simulink model "UAV_Research_Environment"  (R2025a)
settings: Solver=ode23t  StartTime=0.0  StopTime=130  MaxStep=2e-3  RelTol=1e-4  AbsTol=1e-3  EnableMultiTasking=on
InitFcn:
  | skipInitialization = false;
  | 
  | if evalin('base', ...
  |         'exist(''CONTROLLER_TUNING_ACTIVE'',''var'')')
  | 
  |     skipInitialization = evalin('base', ...
  |         'logical(CONTROLLER_TUNING_ACTIVE)');
  | end
  | 
  | if ~skipInitialization
  | 
  |     icraControllerPrepared = false;
  | 
  |     hasICRAVariables = evalin('base', ...
  |         ['exist(''AUTOPILOT'',''var'') && ' ...
  |          'exist(''ICRA_ACTIVE_CONTROLLER'',''var'') && ' ...
  |          'exist(''ICRA_ACTIVE_RUN_ID'',''var'')']);
  | 
  |     if hasICRAVariables
  | 
  |         icraControllerPrepared = evalin('base', ...
  |             ['isstruct(AUTOPILOT) && ' ...
  |              'isfield(AUTOPILOT,''info'') && ' ...
  |              'isfield(AUTOPILOT.info,''ICRAControllerID'') && ' ...
  |              'strcmp(string(AUTOPILOT.info.ICRAControllerID), ' ...
  |                     'string(ICRA_ACTIVE_CONTROLLER))']);
  | 
  |     end
  | 
  |     if icraControllerPrepared
  |         skipInitialization = true;
  |     end
  | end
  | 
  | if ~skipInitialization
  | 
  |     mdl = bdroot;
  | 
  |     mdl_file = get_param(mdl, 'FileName');
  | 
  |     project_root = fileparts(mdl_file);
  | 
  |     init_file = fullfile(project_root, 'initialize_project.m');
  | 
  |     if exist(init_file, 'file')
  | 
  |         run(init_file);
  | 
  |     else
  | 
  |         error('initialize_project.m was not found in the model folder.');
  | 
  |     end
  | end
values from neighbouring files (symbols this model uses):
  A_UAV = struct()    [UAV_analytical.m]
  AUTOPILOT = struct()    [UAV_autopilot.m]
  B_UAV = struct()    [UAV_block.m]
  D = A_UAV.source.propeller_diameter_m    [UAV_analytical.m]    (also in plot_controller_results.m = permute(                  D,                  order); plot_estimator_results.m = permute(              D,              order); plot_mission_results.m = permute(                  D,                  order); plot_touchdown_diagnostics.m = permute(                  D,                  order))
  OPERATOR_MODE = OPERATOR_MODE_MANUAL    [initialize_project.m]    (also in uav_remote_gui.m = uint8(0))
  P_ENV = struct()    [Environment.m]
  P_UAV = struct()    [UAV_simscape.m]
  s = sin(angle)    [uav_remote_gui.m]
  SENSOR = struct()    [UAV_sensors.m]
  TRAJECTORY_CONFIG = struct()    [UAV_trajectories.m]
  TRAJECTORY_ID = uint8(          trajectoryIDNumeric)    [UAV_trajectories.m]
  X = reshape(                  D,                  nt,                  [])    [plot_controller_results.m]    (also in plot_estimator_results.m = reshape(              D,              nt,              []); plot_mission_results.m; plot_touchdown_diagnostics.m; plot_trajectory_3d.m)
  Y = absolutePlanNED(1,:)    [plot_trajectory_3d.m]    (also in uav_remote_gui.m = positionNED(:,1))
  Z = landedCGDown -          absolutePlanNED(3,:)    [plot_trajectory_3d.m]    (also in uav_remote_gui.m = landedCGDown-positionNED(:,3))
undefined symbols (not defined in the file or in its folder): Acceleration_ref, F, fractalcoef, Light, MIL, Position_ref, Velocity_ref, Yaw_ref, YawRate_ref
libraries: sm_lib x49, nesl_utility x29, fl_lib x17, slpidlib x16, simulink x14, ee_lib x5, sdl_lib x4, aerolibwind2 x3, aerolibatmos2 x2, sensorbarometerlib x1, sensorgpslib x1, mspsensorlib x1
(part 7 of 9)

== system UAV_Research_Environment/UAV Plant/UAV Physical [Simscape]/Motor ESC 3/Speed PI Control ==
  wCmd : Inport
  w : Inport  Port=2
  Gain : Gain  Gain=-1
  PI Controller : slpidlib/PID Controller  Controller=PI  Form=Parallel  TimeDomain=Continuous-time  UseExternalTs=off  SampleTime=-1  IntegratorMethod=Forward Euler  FilterMethod=Forward Euler  ControllerParametersSource=internal  P=P_UAV.drive.speed_pi.Kp  I=P_UAV.drive.speed_pi.Ki  UseKiTs=off  D=0.000001  UseExternalDerivativeSource=off  N=10000  UseFilter=on  TunerSelectOption=Transfer Function Based (PID Tuner App)  InitialConditionSource=internal  InitialConditionForIntegrator=0  InitialConditionForFilter=0  DifferentiatorICPrevScaledInput=0  ExternalReset=none  TrackingMode=off  Kt=1  LimitOutput=on  SatLimitsSource=internal  UpperSaturationLimit=P_UAV.drive.speed_pi.torque_limit_Nm  LowerSaturationLimit=-P_UAV.drive.speed_pi.torque_limit_Nm  LinearizeAsGain=on  AntiWindupMode=clamping  Kb=1  LimitIntegrator=off  UpperIntegratorSaturationLimit=inf  LowerIntegratorSaturationLimit=-inf  POutMin=[]  POutMax=[]  IOutMin=[]  IOutMax=[]  DOutMin=[]  DOutMax=[]  NOutMin=[]  NOutMax=[]  SumOutMin=[]  SumOutMax=[]  SaturationOutMin=[]  SaturationOutMax=[]  PParamMin=[]  PParamMax=[]  IParamMin=[]  IParamMax=[]  DParamMin=[]  DParamMax=[]  NParamMin=[]  NParamMax=[]  KbParamMin=[]  KbParamMax=[]  KtParamMin=[]  KtParamMax=[]  KbOutMin=[]  KbOutMax=[]  KtOutMin=[]  KtOutMax=[]  IntegratorOutMin=[]  IntegratorOutMax=[]  FilterOutMin=[]  FilterOutMax=[]  SumI1OutMin=[]  SumI1OutMax=[]  SumI2OutMin=[]  SumI2OutMax=[]  SumI3OutMin=[]  SumI3OutMax=[]  SumI4OutMin=[]  SumI4OutMax=[]  SumDOutMin=[]  SumDOutMax=[]  DifferentiatorOutMin=[]  DifferentiatorOutMax=[]  FilterDiffOutCoefMin=[]  FilterDiffOutCoefMax=[]  ReciprocalOutMin=[]  ReciprocalOutMax=[]  SumDenOutMin=[]  SumDenOutMax=[]  SumNumOutMin=[]  SumNumOutMax=[]  DivideOutMin=[]  DivideOutMax=[]  UdiffTsProdOutMin=[]  UdiffTsProdOutMax=[]  NTsProdOutMin=[]  NTsProdOutMax=[]  UintegralTsProdOutMin=[]  UintegralTsProdOutMax=[]  UngainTsProdOutMin=[]  UngainTsProdOutMax=[]  ClampingZeroOutDataTypeStr=Inherit: Inherit via back propagation  ClampingZeroOutMin=[]  ClampingZeroOutMax=[]  FilterDenConstantOutDataTypeStr=Inherit: Inherit via back propagation  FilterDenConstantOutMin=[]  FilterDenConstantOutMax=[]  PCopyOutDataTypeStr=Inherit: Inherit via back propagation  PCopyOutMin=[]  PCopyOutMax=[]  NCopyOutDataTypeStr=Inherit: Inherit via back propagation  NCopyOutMin=[]  NCopyOutMax=[]  IntegratorContinuousStateAttributes=''  IntegratorStateMustResolveToSignalObject=off  IntegratorRTWStateStorageClass=Auto  FilterContinuousStateAttributes=''  FilterStateMustResolveToSignalObject=off  FilterRTWStateStorageClass=Auto  ParallelPVariant=InternalParameters  IdealPVariant=Disabled  IVariant=InternalParameters  DVariant=Disabled  IntegratorVariant=Continuous  SatVariant=Enabled  AWVariant=ContClampingParallel  PCopyVariant=Disabled  TRVariant=Disabled  FdbkBlocksVariant=Forward  IdealPFdbkVariant=Disabled  SatFdbkVariant=Disabled  DerivativeFilterVariant=Disabled  NVariant=Disabled  NCopyVariant=Disabled_SignalSpec  FilterICVariant=Disabled  IntegratorICVariant=InternalICs  ExternalResetVariant=Disabled  TRSumVariant=Passthrough  SumFdbkVariant=Disabled  SumVariant=Sum_PI  TsampFilterVariant=InternalTs  TsampNgainVariant=Passthrough  TsampIntegralVariant=Disabled_SignalSpec  ExternalSaturationOutDataTypeStr=Inherit: Same as second input  DerivativeSourceVariant=Disabled  PreIntVariant=InternalPreInt
  Sum : Sum  Inputs=|+-
  TorqueCmd : Outport
  wires:
  wCmd/1 -> Gain/1
  Sum/1 -> PI Controller/1  "rad/s"
  w/1 -> Sum/2
  PI Controller/1 -> TorqueCmd/1  "N*m"
  Gain/1 -> Sum/1

== system UAV_Research_Environment/UAV Plant/UAV Physical [Simscape]/Motor ESC 4/Speed PI Control ==
  wCmd : Inport
  w : Inport  Port=2
  Gain : Gain  Gain=-1
  PI Controller : slpidlib/PID Controller  Controller=PI  Form=Parallel  TimeDomain=Continuous-time  UseExternalTs=off  SampleTime=-1  IntegratorMethod=Forward Euler  FilterMethod=Forward Euler  ControllerParametersSource=internal  P=P_UAV.drive.speed_pi.Kp  I=P_UAV.drive.speed_pi.Ki  UseKiTs=off  D=0.000001  UseExternalDerivativeSource=off  N=10000  UseFilter=on  TunerSelectOption=Transfer Function Based (PID Tuner App)  InitialConditionSource=internal  InitialConditionForIntegrator=0  InitialConditionForFilter=0  DifferentiatorICPrevScaledInput=0  ExternalReset=none  TrackingMode=off  Kt=1  LimitOutput=on  SatLimitsSource=internal  UpperSaturationLimit=P_UAV.drive.speed_pi.torque_limit_Nm  LowerSaturationLimit=-P_UAV.drive.speed_pi.torque_limit_Nm  LinearizeAsGain=on  AntiWindupMode=clamping  Kb=1  LimitIntegrator=off  UpperIntegratorSaturationLimit=inf  LowerIntegratorSaturationLimit=-inf  POutMin=[]  POutMax=[]  IOutMin=[]  IOutMax=[]  DOutMin=[]  DOutMax=[]  NOutMin=[]  NOutMax=[]  SumOutMin=[]  SumOutMax=[]  SaturationOutMin=[]  SaturationOutMax=[]  PParamMin=[]  PParamMax=[]  IParamMin=[]  IParamMax=[]  DParamMin=[]  DParamMax=[]  NParamMin=[]  NParamMax=[]  KbParamMin=[]  KbParamMax=[]  KtParamMin=[]  KtParamMax=[]  KbOutMin=[]  KbOutMax=[]  KtOutMin=[]  KtOutMax=[]  IntegratorOutMin=[]  IntegratorOutMax=[]  FilterOutMin=[]  FilterOutMax=[]  SumI1OutMin=[]  SumI1OutMax=[]  SumI2OutMin=[]  SumI2OutMax=[]  SumI3OutMin=[]  SumI3OutMax=[]  SumI4OutMin=[]  SumI4OutMax=[]  SumDOutMin=[]  SumDOutMax=[]  DifferentiatorOutMin=[]  DifferentiatorOutMax=[]  FilterDiffOutCoefMin=[]  FilterDiffOutCoefMax=[]  ReciprocalOutMin=[]  ReciprocalOutMax=[]  SumDenOutMin=[]  SumDenOutMax=[]  SumNumOutMin=[]  SumNumOutMax=[]  DivideOutMin=[]  DivideOutMax=[]  UdiffTsProdOutMin=[]  UdiffTsProdOutMax=[]  NTsProdOutMin=[]  NTsProdOutMax=[]  UintegralTsProdOutMin=[]  UintegralTsProdOutMax=[]  UngainTsProdOutMin=[]  UngainTsProdOutMax=[]  ClampingZeroOutDataTypeStr=Inherit: Inherit via back propagation  ClampingZeroOutMin=[]  ClampingZeroOutMax=[]  FilterDenConstantOutDataTypeStr=Inherit: Inherit via back propagation  FilterDenConstantOutMin=[]  FilterDenConstantOutMax=[]  PCopyOutDataTypeStr=Inherit: Inherit via back propagation  PCopyOutMin=[]  PCopyOutMax=[]  NCopyOutDataTypeStr=Inherit: Inherit via back propagation  NCopyOutMin=[]  NCopyOutMax=[]  IntegratorContinuousStateAttributes=''  IntegratorStateMustResolveToSignalObject=off  IntegratorRTWStateStorageClass=Auto  FilterContinuousStateAttributes=''  FilterStateMustResolveToSignalObject=off  FilterRTWStateStorageClass=Auto  ParallelPVariant=InternalParameters  IdealPVariant=Disabled  IVariant=InternalParameters  DVariant=Disabled  IntegratorVariant=Continuous  SatVariant=Enabled  AWVariant=ContClampingParallel  PCopyVariant=Disabled  TRVariant=Disabled  FdbkBlocksVariant=Forward  IdealPFdbkVariant=Disabled  SatFdbkVariant=Disabled  DerivativeFilterVariant=Disabled  NVariant=Disabled  NCopyVariant=Disabled_SignalSpec  FilterICVariant=Disabled  IntegratorICVariant=InternalICs  ExternalResetVariant=Disabled  TRSumVariant=Passthrough  SumFdbkVariant=Disabled  SumVariant=Sum_PI  TsampFilterVariant=InternalTs  TsampNgainVariant=Passthrough  TsampIntegralVariant=Disabled_SignalSpec  ExternalSaturationOutDataTypeStr=Inherit: Same as second input  DerivativeSourceVariant=Disabled  PreIntVariant=InternalPreInt
  Sum : Sum  Inputs=|+-
  TorqueCmd : Outport
  wires:
  Sum/1 -> PI Controller/1  "rad/s"
  w/1 -> Sum/2
  PI Controller/1 -> TorqueCmd/1  "N*m"
  Gain/1 -> Sum/1
  wCmd/1 -> Gain/1

== system UAV_Research_Environment/Autopilot/Flight Control/Main Controller/Horizontal Velocity Control/Subsystem ==
  CmdAcceleration_BodyXY : Inport
  Constant1 : Constant  Value=AUTOPILOT.horizontal.maxTilt_rad
  Constant2 : Constant  Value=-AUTOPILOT.horizontal.maxTilt_rad
  Gain : Gain  Gain=-1
  Gain1 : Gain  Gain=1 / AUTOPILOT.gravity.magnitude_m_s2
  Mux1 : Mux  Inputs=2
  Saturation Dynamic1 : simulink/Discontinuities/Saturation Dynamic  OutMin=[]  OutMax=[]  OutDataTypeStr=Inherit: Same as second input  OutDataType=fixdt(1, 16)  OutScaling=2^-10  DoSatur=off
  Selector2 : Selector  InputPortWidth=2  IndexOptions=Index vector (dialog)  Indices=1  OutputSizes=1
  Selector3 : Selector  InputPortWidth=2  IndexOptions=Index vector (dialog)  Indices=2  OutputSizes=1
  Trigonometric Function : Trigonometry  Operator=atan
  y : Outport
  wires:
  Trigonometric Function/1 -> Saturation Dynamic1/2  "CmdAttitude_raw"
  Mux1/1 -> Gain1/1
  Saturation Dynamic1/1 -> y/1
  Gain/1 -> Mux1/2  "MinusAx_cmd"
  CmdAcceleration_BodyXY/1 -> Selector3/1, Selector2/1
  Selector2/1 -> Gain/1  "Ax_cmd"
  Constant2/1 -> Saturation Dynamic1/3
  Gain1/1 -> Trigonometric Function/1
  Selector3/1 -> Mux1/1  "Ay_cmd"
  Constant1/1 -> Saturation Dynamic1/1

== matlab function UAV_Research_Environment/UAV Plant/UAV Analytical [ODEs]/Attitude Kinematics/Quaternion Kinematics ==
  data: Omega_body input; Q_dot output; Q input
function Q_dot = Quaternion_Kinematics(Omega_body,Q)

p = Omega_body(1);

q = Omega_body(2);

r = Omega_body(3);

Q_dot = 0.5 * [ ...
     0, -p, -q, -r; ...
     p,  0,  r, -q; ...
     q, -r,  0,  p; ...
     r,  q, -p,  0] * Q;

end

== matlab function UAV_Research_Environment/UAV Plant/UAV Analytical [ODEs]/Attitude Kinematics/Normalize Quaternion ==
  data: Q_raw input; Q output
function Q = Normalize_Quaternion(Q_raw)
%#codegen

n = sqrt(sum(Q_raw.^2));

if n > eps
    Q = Q_raw / n;
else
    Q = [1;0;0;0];
end

end

== matlab function UAV_Research_Environment/Live Telemetry/Telemetry_Pack ==
  data: t input; Telemetry output; Phase input; Active input; Complete input; Position_ref input; mode input; armed input; missionComplete input; Landed input; Position input; Euler input; MotorSpeeds input; MissionPlan input; TruePosition input; TrueEuler input; EstPosition input; NumWaypoints input
function Telemetry = Telemetry_Pack( ...
    t, ...
    Phase, ...
    Active, ...
    Complete, ...
    Position_ref, ...
    mode, ...
    armed, ...
    missionComplete, ...
    Landed, ...
    Position, ...
    Euler, ...
    MotorSpeeds, ...
    MissionPlan, ...
    TruePosition, ...
    TrueEuler, ...
    EstPosition, ...
    NumWaypoints)
maxWaypoints = ...
    size( ...
        MissionPlan, ...
        2);
genericTelemetryLength = ...
    59 + ...
    4*maxWaypoints;
Telemetry = ...
    zeros( ...
        genericTelemetryLength, ...
        1);
positionRefValid = ...
    numel(Position_ref) >= 3;
operationalPositionValid = ...
    numel(Position) >= 3;
operationalEulerValid = ...
    numel(Euler) >= 3;
motorSpeedsValid = ...
    numel(MotorSpeeds) >= 4;
truePositionValid = ...
    numel(TruePosition) >= 3;
trueEulerValid = ...
    numel(TrueEuler) >= 3;
estPositionValid = ...
    numel(EstPosition) >= 3;
missionPlanDimensionsValid = ...
    size(MissionPlan,1) == 4 && ...
    maxWaypoints >= 1;
numWaypointsRaw = ...
    double( ...
        NumWaypoints);
numWaypointsValid = ...
    isscalar(numWaypointsRaw) && ...
    isfinite(numWaypointsRaw) && ...
    numWaypointsRaw >= 1 && ...
    numWaypointsRaw <= maxWaypoints && ...
    abs( ...
        numWaypointsRaw - ...
        round(numWaypointsRaw)) < 1.0e-12;
if numWaypointsValid
    activeNumWaypoints = ...
        round( ...
            numWaypointsRaw);
else
    activeNumWaypoints = ...
        0.0;
end
Telemetry(1) = ...
    finiteScalarOrZero( ...
        t);
Telemetry(2) = ...
    finiteScalarOrZero( ...
        Phase);
Telemetry(3) = ...
    finiteScalarOrZero( ...
        Active);
Telemetry(4) = ...
    finiteScalarOrZero( ...
        Complete);
Telemetry(5) = ...
    finiteScalarOrZero( ...
        mode);
Telemetry(6) = ...
    finiteScalarOrZero( ...
        armed);
Telemetry(7) = ...
    finiteScalarOrZero( ...
        missionComplete);
Telemetry(8) = ...
    finiteScalarOrZero( ...
        Landed);
if positionRefValid
    Telemetry(9) = ...
        finiteScalarOrZero( ...
            Position_ref(1));
    Telemetry(10) = ...
        finiteScalarOrZero( ...
            Position_ref(2));
    Telemetry(11) = ...
        finiteScalarOrZero( ...
            Position_ref(3));
end
if operationalPositionValid
    Telemetry(12) = ...
        finiteScalarOrZero( ...
            Position(1));
    Telemetry(13) = ...
        finiteScalarOrZero( ...
            Position(2));
    Telemetry(14) = ...
        finiteScalarOrZero( ...
            Position(3));
end
legacyWaypointSlots = ...
    7;
if missionPlanDimensionsValid
    for k = 1:legacyWaypointSlots
        if k <= maxWaypoints
            Telemetry(14 + k) = ...
                finiteScalarOrZero( ...
                    MissionPlan(1,k));
            Telemetry(21 + k) = ...
                finiteScalarOrZero( ...
                    MissionPlan(2,k));
            Telemetry(28 + k) = ...
                finiteScalarOrZero( ...
                    MissionPlan(3,k));
            Telemetry(35 + k) = ...
                finiteScalarOrZero( ...
                    MissionPlan(4,k));
        end
    end
end
if operationalEulerValid
    Telemetry(43) = ...
        finiteScalarOrZero( ...
            Euler(1));
    Telemetry(44) = ...
        finiteScalarOrZero( ...
            Euler(2));
    Telemetry(45) = ...
        finiteScalarOrZero( ...
            Euler(3));
end
if motorSpeedsValid
    Telemetry(46) = ...
        finiteScalarOrZero( ...
            MotorSpeeds(1));
    Telemetry(47) = ...
        finiteScalarOrZero( ...
            MotorSpeeds(2));
    Telemetry(48) = ...
        finiteScalarOrZero( ...
            MotorSpeeds(3));
    Telemetry(49) = ...
        finiteScalarOrZero( ...
            MotorSpeeds(4));
end
if truePositionValid
    Telemetry(50) = ...
        finiteScalarOrZero( ...
            TruePosition(1));
    Telemetry(51) = ...
        finiteScalarOrZero( ...
            TruePosition(2));
    Telemetry(52) = ...
        finiteScalarOrZero( ...
            TruePosition(3));
end
if trueEulerValid
    Telemetry(53) = ...
        finiteScalarOrZero( ...
            TrueEuler(1));
    Telemetry(54) = ...
        finiteScalarOrZero( ...
            TrueEuler(2));
    Telemetry(55) = ...
        finiteScalarOrZero( ...
            TrueEuler(3));
end
if estPositionValid
    Telemetry(56) = ...
        finiteScalarOrZero( ...
            EstPosition(1));
    Telemetry(57) = ...
        finiteScalarOrZero( ...
            EstPosition(2));
    Telemetry(58) = ...
        finiteScalarOrZero( ...
            EstPosition(3));
end
Telemetry(59) = ...
    double( ...
        activeNumWaypoints);
northStartIndex = ...
    60;
eastStartIndex = ...
    60 + ...
    maxWaypoints;
downStartIndex = ...
    60 + ...
    2*maxWaypoints;
yawStartIndex = ...
    60 + ...
    3*maxWaypoints;
if missionPlanDimensionsValid && ...
        numWaypointsValid
    for k = 1:maxWaypoints
        if k <= activeNumWaypoints
            Telemetry( ...
                northStartIndex + k - 1) = ...
                finiteScalarOrZero( ...
                    MissionPlan(1,k));
            Telemetry( ...
                eastStartIndex + k - 1) = ...
                finiteScalarOrZero( ...
                    MissionPlan(2,k));
            Telemetry( ...
                downStartIndex + k - 1) = ...
                finiteScalarOrZero( ...
                    MissionPlan(3,k));
            Telemetry( ...
                yawStartIndex + k - 1) = ...
                finiteScalarOrZero( ...
                    MissionPlan(4,k));
        end
    end
end
end
function valueOut = finiteScalarOrZero(valueIn)
valueOut = ...
    double( ...
        valueIn);
if ~isfinite(valueOut)
    valueOut = ...
        0.0;
end
end

== stateflow chart UAV_Research_Environment/Autopilot/Flight Management/Mode Logic ==
  state Disarmed
    entry:
    mode = 1;
    armed = false;
    reset = true;
    missionComplete = false;
  state ArmedIdle
    entry:
    mode = 2;
    armed = true;
    reset = false;
    missionComplete = false;
  state TrajectoryMode
    entry:
    mode = 6;
    armed = true;
    reset = false;
    missionComplete = false;
  state LandingHold
    entry:
    mode = 6;
    armed = true;
    reset = false;
    missionComplete = true;
  state NavFailsafe
    entry:
    mode = 7;
    armed = true;
    reset = false;
    missionComplete = false;
  state FailsafeLanded
    entry:
    mode = 2;
    armed = true;
    reset = false;
    missionComplete = false;
  state TouchdownSettle
    entry:
    mode = 2;
    armed = true;
    reset = false;
    missionComplete = true;
  state LandedArmed
    entry:
    mode = 2;
    armed = true;
    reset = false;
    missionComplete = true;
  (default) -> Disarmed : {lastRunRequestID = uint32(0);}
  ArmedIdle -> TrajectoryMode [order 2] : [NavValid && RunTrajectoryRequestID ~= lastRunRequestID]
      | {lastRunRequestID = RunTrajectoryRequestID;}
  Disarmed -> ArmedIdle : [ArmCommand && NavValid]
  ArmedIdle -> Disarmed [order 1] : [~ArmCommand]
  TrajectoryMode -> Disarmed [order 1] : [~ArmCommand]
  LandedArmed -> TrajectoryMode [order 2] : [NavValid && RunTrajectoryRequestID ~= lastRunRequestID]
      | {lastRunRequestID = RunTrajectoryRequestID;}
  TrajectoryMode -> NavFailsafe [order 2] : [~NavValid]
  TrajectoryMode -> LandingHold [order 3] : [Complete]
  LandedArmed -> Disarmed [order 1] : [~ArmCommand]
  TouchdownSettle -> Disarmed [order 2] : [~ArmCommand]
  FailsafeLanded -> Disarmed : [~ArmCommand]
  NavFailsafe -> Disarmed [order 2] : [~ArmCommand]
  LandingHold -> Disarmed [order 1] : [~ArmCommand]
  LandingHold -> NavFailsafe [order 2] : [~NavValid]
  LandingHold -> TouchdownSettle [order 3] : [TouchdownCandidate]
  NavFailsafe -> FailsafeLanded [order 1] : [Landed]
  TouchdownSettle -> LandedArmed [order 1] : [Landed]
  data: mode output double size=1; armed output boolean size=1; reset output boolean size=1; missionComplete output boolean size=1; Complete input boolean; ArmCommand input boolean; RunTrajectoryRequestID input uint32; lastRunRequestID local uint32; Landed input boolean; TouchdownCandidate input boolean size=1; NavValid input boolean size=1

== matlab function UAV_Research_Environment/Autopilot/Flight Control/Error Computation/Wrap Yaw Error ==
  data: YawErrorRaw input; YawError output
function YawError = Wrap_Yaw_Error(YawErrorRaw)
%#codegen

YawError = atan2( ...
    sin(YawErrorRaw), ...
    cos(YawErrorRaw));

end

== matlab function UAV_Research_Environment/UAV Plant/UAV Analytical [ODEs]/Ground Contact/Ground_Contact_Model ==
  data: p_ned input; F_ground_body output; v_ned input; R_BN input; Omega_body input; Tau_ground_body output; UAV_CONTACT parameter
function [F_ground_body, Tau_ground_body] = ...
    Ground_Contact_Model( ...
        p_ned, ...
        v_ned, ...
        R_BN, ...
        Omega_body, ...
        UAV_CONTACT)
F_ground_body = ...
    zeros(3,1);
Tau_ground_body = ...
    zeros(3,1);
kGround = ...
    UAV_CONTACT.stiffness_N_m;
cGround = ...
    UAV_CONTACT.damping_N_s_m;
muStatic = ...
    UAV_CONTACT.static_friction;
muDynamic = ...
    UAV_CONTACT.dynamic_friction;
vCritical = ...
    UAV_CONTACT.critical_velocity_m_s;
if vCritical < 1e-6
    vCritical = ...
        1e-6;
end
groundDown = ...
    UAV_CONTACT.ground_down_m;
for i = 1:4
    r_body = [ ...
        UAV_CONTACT.arm_body_m(i,1);
        UAV_CONTACT.arm_body_m(i,2);
        UAV_CONTACT.arm_body_m(i,3)];
    r_ned = ...
        R_BN * r_body;
    p_contact_ned = ...
        p_ned + r_ned;
    v_rot_body = ...
        cross( ...
            Omega_body, ...
            r_body);
    v_rot_ned = ...
        R_BN * v_rot_body;
    v_contact_ned = ...
        v_ned + ...
        v_rot_ned;
    penetration = ...
        p_contact_ned(3) - ...
        groundDown;
    if penetration > 0.0
        penetrationRate = ...
            v_contact_ned(3);
        normalForce = ...
            kGround * penetration + ...
            cGround * penetrationRate;
        if normalForce < 0.0
            normalForce = ...
                0.0;
        end
        vNorth = ...
            v_contact_ned(1);
        vEast = ...
            v_contact_ned(2);
        tangentialSpeed = ...
            sqrt( ...
                vNorth*vNorth + ...
                vEast*vEast);
        velocityRatio = ...
            tangentialSpeed / ...
            vCritical;
        mu = ...
            muDynamic + ...
            (muStatic - muDynamic) * ...
            exp( ...
                -(velocityRatio * velocityRatio));
        denominator = ...
            sqrt( ...
                tangentialSpeed*tangentialSpeed + ...
                vCritical*vCritical);
        frictionNorth = ...
           -mu * normalForce * ...
            vNorth / ...
            denominator;
        frictionEast = ...
           -mu * normalForce * ...
            vEast / ...
            denominator;
        F_contact_ned = [ ...
            frictionNorth;
            frictionEast;
           -normalForce];
        F_contact_body = ...
            R_BN.' * ...
            F_contact_ned;
        F_ground_body = ...
            F_ground_body + ...
            F_contact_body;
        Tau_contact_body = ...
            cross( ...
                r_body, ...
                F_contact_body);
        Tau_ground_body = ...
            Tau_ground_body + ...
            Tau_contact_body;
    end
end
end

== matlab function UAV_Research_Environment/Autopilot/Landed Detector/Landing_Confirmation ==
  settings: updateMethod=DISCRETE
  data: Position input size=[3 1]; Landed output size=[1 1]; Velocity input size=[3 1]; Euler input size=[3 1]; AngularRate input size=[3 1]; Position_ref input size=[3 1]; Complete input size=[1 1]; Phase input; RunTrajectoryRequestID input size=[1 1]; NavValid input; TouchdownCandidate output; NumWaypoints input
function [Landed, TouchdownCandidate] = Landing_Confirmation( ...
    Position, ...
    Velocity, ...
    Euler, ...
    AngularRate, ...
    Position_ref, ...
    Complete, ...
    Phase, ...
    RunTrajectoryRequestID, ...
    NavValid, ...
    NumWaypoints)

persistent lastRunRequestID
persistent touchdownCounter
persistent touchdownCandidateLatched
persistent confirmationCounter
persistent landedLatched
persistent completeCounter
persistent homePosition
persistent homeInitialized

if isempty(lastRunRequestID)

    lastRunRequestID = ...
        uint32(0);

    touchdownCounter = ...
        uint32(0);

    touchdownCandidateLatched = ...
        false;

    confirmationCounter = ...
        uint32(0);

    landedLatched = ...
        false;

    completeCounter = ...
        uint32(0);

    homePosition = ...
        zeros(3,1);

    homeInitialized = ...
        false;

end

groundDatumAlpha = ...
    0.02;

touchdownAboveGroundTolerance_m = ...
    0.10;

touchdownBelowGroundTolerance_m = ...
    0.15;

touchdownHorizontalSpeedThreshold_m_s = ...
    0.45;

touchdownVerticalSpeedThreshold_m_s = ...
    0.10;

touchdownRollThreshold_rad = ...
    15.0 * pi / 180.0;

touchdownPitchThreshold_rad = ...
    15.0 * pi / 180.0;

touchdownRequiredSamples = ...
    uint32(50);

completeGuardSamples = ...
    uint32(50);

referenceGroundTolerance_m = ...
    0.30;

landedVerticalPositionThreshold_m = ...
    0.15;

landedHorizontalSpeedThreshold_m_s = ...
    0.40;

landedVerticalSpeedThreshold_m_s = ...
    0.10;

landedRollThreshold_rad = ...
    12.0 * pi / 180.0;

landedPitchThreshold_rad = ...
    12.0 * pi / 180.0;

landedAngularRateThreshold_rad_s = ...
    0.60;

landedRequiredSamples = ...
    uint32(100);

requestID = ...
    uint32( ...
        RunTrajectoryRequestID);

navigationValid = ...
    logical( ...
        NavValid);

missionComplete = ...
    logical( ...
        Complete);

phaseRaw = ...
    double( ...
        Phase);

numWaypointsRaw = ...
    double( ...
        NumWaypoints);

positionValid = ...
    isfinite(Position(1)) && ...
    isfinite(Position(2)) && ...
    isfinite(Position(3));

velocityValid = ...
    isfinite(Velocity(1)) && ...
    isfinite(Velocity(2)) && ...
    isfinite(Velocity(3));

eulerValid = ...
    isfinite(Euler(1)) && ...
    isfinite(Euler(2)) && ...
    isfinite(Euler(3));

angularRateValid = ...
    isfinite(AngularRate(1)) && ...
    isfinite(AngularRate(2)) && ...
    isfinite(AngularRate(3));

positionReferenceValid = ...
    isfinite(Position_ref(1)) && ...
    isfinite(Position_ref(2)) && ...
    isfinite(Position_ref(3));

stateDataValid = ...
    positionValid && ...
    velocityValid && ...
    eulerValid && ...
    angularRateValid;

if velocityValid

    vNorth = ...
        Velocity(1);

    vEast = ...
        Velocity(2);

    vDown = ...
        Velocity(3);

    horizontalSpeed = ...
        sqrt( ...
            vNorth*vNorth + ...
            vEast*vEast);

    verticalSpeed = ...
        abs( ...
            vDown);

else

    vNorth = ...
        0.0;

    vEast = ...
        0.0;

    vDown = ...
        0.0;

    horizontalSpeed = ...
        Inf;

    verticalSpeed = ...
        Inf;

end

if eulerValid

    roll = ...
        Euler(1);

    pitch = ...
        Euler(2);

else

    roll = ...
        0.0;

    pitch = ...
        0.0;

end

if requestID == uint32(0) && ...
        positionValid

    currentPosition = ...
        reshape( ...
            Position, ...
            3, ...
            1);

    if ~homeInitialized

        homePosition = ...
            currentPosition;

        homeInitialized = ...
            true;

    else

        homePosition = ...
            (1.0 - groundDatumAlpha) * ...
            homePosition + ...
            groundDatumAlpha * ...
            currentPosition;

    end

end

if requestID ~= lastRunRequestID

    lastRunRequestID = ...
        requestID;

    touchdownCounter = ...
        uint32(0);

    touchdownCandidateLatched = ...
        false;

    confirmationCounter = ...
        uint32(0);

    landedLatched = ...
        false;

    completeCounter = ...
        uint32(0);

    if ~homeInitialized && ...
            requestID > uint32(0) && ...
            positionValid

        homePosition = ...
            reshape( ...
                Position, ...
                3, ...
                1);

        homeInitialized = ...
            true;

    end

end

phaseValid = ...
    isscalar(phaseRaw) && ...
    isfinite(phaseRaw);

numWaypointsValid = ...
    isscalar(numWaypointsRaw) && ...
    isfinite(numWaypointsRaw) && ...
    numWaypointsRaw >= 3.0;

if phaseValid

    currentPhase = ...
        round( ...
            phaseRaw);

else

    currentPhase = ...
        -1.0;

end

if numWaypointsValid

    activeNumWaypoints = ...
        round( ...
            numWaypointsRaw);

    landingPhase = ...
        2.0 * ...
        activeNumWaypoints - ...
        3.0;

    completePhase = ...
        2.0 * ...
        activeNumWaypoints - ...
        2.0;

else

    activeNumWaypoints = ...
        0.0;

    landingPhase = ...
        Inf;

    completePhase = ...
        Inf;

end

landingPhaseActive = ...
    phaseValid && ...
    numWaypointsValid && ...
    currentPhase == landingPhase;

completePhaseActive = ...
    phaseValid && ...
    numWaypointsValid && ...
    currentPhase == completePhase;

if requestID > uint32(0) && ...
        missionComplete

    if completeCounter < completeGuardSamples

        completeCounter = ...
            completeCounter + ...
            uint32(1);

    end

else

    completeCounter = ...
        uint32(0);

end

completeConfirmed = ...
    missionComplete && ...
    completeCounter >= ...
    completeGuardSamples;

if homeInitialized && ...
        positionValid

    groundDown = ...
        homePosition(3);

    groundVerticalSignedError = ...
        Position(3) - ...
        groundDown;

    groundVerticalError = ...
        abs( ...
            groundVerticalSignedError);

    touchdownNearGround = ...
        groundVerticalSignedError >= ...
            -touchdownAboveGroundTolerance_m && ...
        groundVerticalSignedError <= ...
            touchdownBelowGroundTolerance_m;

    landedNearGround = ...
        groundVerticalError <= ...
        landedVerticalPositionThreshold_m;

else

    groundDown = ...
        0.0;

    groundVerticalSignedError = ...
        Inf;

    groundVerticalError = ...
        Inf;

    touchdownNearGround = ...
        false;

    landedNearGround = ...
        false;

end

if homeInitialized && ...
        positionReferenceValid

    referenceGroundError = ...
        abs( ...
            Position_ref(3) - ...
            groundDown);

    referenceNearGround = ...
        referenceGroundError <= ...
        referenceGroundTolerance_m;

else

    referenceGroundError = ...
        Inf;

    referenceNearGround = ...
        false;

end

touchdownLowHorizontalSpeed = ...
    horizontalSpeed <= ...
    touchdownHorizontalSpeedThreshold_m_s;

touchdownLowVerticalSpeed = ...
    verticalSpeed <= ...
    touchdownVerticalSpeedThreshold_m_s;

if eulerValid

    touchdownLevelRoll = ...
        abs(roll) <= ...
        touchdownRollThreshold_rad;

    touchdownLevelPitch = ...
        abs(pitch) <= ...
        touchdownPitchThreshold_rad;

    touchdownLevelAttitude = ...
        touchdownLevelRoll && ...
        touchdownLevelPitch;

else

    touchdownLevelAttitude = ...
        false;

end

touchdownPhysicalCondition = ...
    stateDataValid && ...
    homeInitialized && ...
    touchdownNearGround && ...
    touchdownLowHorizontalSpeed && ...
    touchdownLowVerticalSpeed && ...
    touchdownLevelAttitude;

normalTouchdownCandidate = ...
    requestID > uint32(0) && ...
    completeConfirmed && ...
    referenceNearGround && ...
    touchdownPhysicalCondition;

failsafeTouchdownCandidate = ...
    requestID > uint32(0) && ...
    ~navigationValid && ...
    touchdownPhysicalCondition;

touchdownCandidateRaw = ...
    normalTouchdownCandidate || ...
    failsafeTouchdownCandidate;

if ~touchdownCandidateLatched

    if touchdownCandidateRaw

        if touchdownCounter < touchdownRequiredSamples

            touchdownCounter = ...
                touchdownCounter + ...
                uint32(1);

        end

        if touchdownCounter >= touchdownRequiredSamples

            touchdownCandidateLatched = ...
                true;

        end

    else

        touchdownCounter = ...
            uint32(0);

    end

end

landedLowHorizontalSpeed = ...
    horizontalSpeed <= ...
    landedHorizontalSpeedThreshold_m_s;

landedLowVerticalSpeed = ...
    verticalSpeed <= ...
    landedVerticalSpeedThreshold_m_s;

if eulerValid

    landedLevelRoll = ...
        abs(roll) <= ...
        landedRollThreshold_rad;

    landedLevelPitch = ...
        abs(pitch) <= ...
        landedPitchThreshold_rad;

    landedLevelAttitude = ...
        landedLevelRoll && ...
        landedLevelPitch;

else

    landedLevelAttitude = ...
        false;

end

if angularRateValid

    p = ...
        AngularRate(1);

    q = ...
        AngularRate(2);

    r = ...
        AngularRate(3);

    angularRateMagnitude = ...
        sqrt( ...
            p*p + ...
            q*q + ...
            r*r);

else

    angularRateMagnitude = ...
        Inf;

end

landedLowAngularRate = ...
    angularRateMagnitude <= ...
    landedAngularRateThreshold_rad_s;

physicallyStable = ...
    stateDataValid && ...
    homeInitialized && ...
    landedNearGround && ...
    landedLowHorizontalSpeed && ...
    landedLowVerticalSpeed && ...
    landedLevelAttitude && ...
    landedLowAngularRate;

normalLandingCandidate = ...
    requestID > uint32(0) && ...
    ( ...
        touchdownCandidateLatched || ...
        missionComplete || ...
        completePhaseActive ...
    ) && ...
    physicallyStable;

failsafeLandingCandidate = ...
    requestID > uint32(0) && ...
    ~navigationValid && ...
    physicallyStable;

landingCandidate = ...
    normalLandingCandidate || ...
    failsafeLandingCandidate;

if ~landedLatched

    if landingCandidate

        if confirmationCounter < landedRequiredSamples

            confirmationCounter = ...
                confirmationCounter + ...
                uint32(1);

        end

        if confirmationCounter >= landedRequiredSamples

            landedLatched = ...
                true;

        end

    else

        confirmationCounter = ...
            uint32(0);

    end

end

if landedLatched

    touchdownCandidateLatched = ...
        true;

end

Landed = ...
    landedLatched;

TouchdownCandidate = ...
    touchdownCandidateLatched;

end
